simulink model "UIMUFSLR"  (R2022b)
settings: Solver=VariableStepAuto  StartTime=0.0  StopTime=10  RelTol=1e-3
values from neighbouring files (symbols this model uses):
  B1 = full(B{1,1})    [load_simulink_inputdata.m]
  B2 = full(B{1,2})    [load_simulink_inputdata.m]
  C1 = full(C{1,1})    [load_simulink_inputdata.m]
  C2 = full(C{1,2})    [load_simulink_inputdata.m]
  D1 = full(D{1,1})    [load_simulink_inputdata.m]
  D2 = full(D{1,2})    [load_simulink_inputdata.m]
  S1 = full(S{1,1})    [load_simulink_inputdata.m]
  S2 = full(S{1,2})    [load_simulink_inputdata.m]
  SC = SC + S{i}    [load_simulink_inputdata.m]
  XX1 = full(XX{1,1})    [load_simulink_inputdata.m]
  XX2 = full(XX{1,2})    [load_simulink_inputdata.m]
  Y = YT'    [load_simulink_inputdata.m]
undefined symbols (not defined in the file or in its folder): para
settings Model: Creator=86135  LastModifiedBy=86135

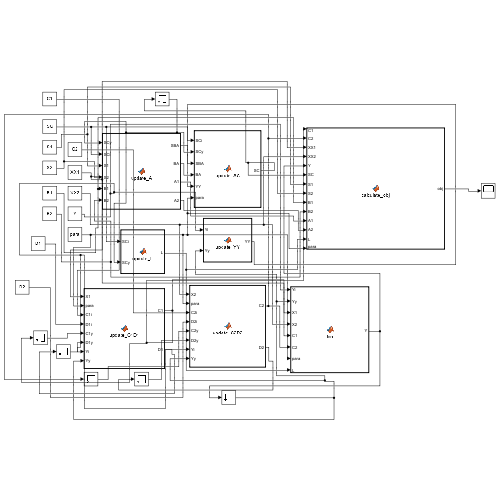
[thumbnail: Simulink's stored preview of the top-level diagram]
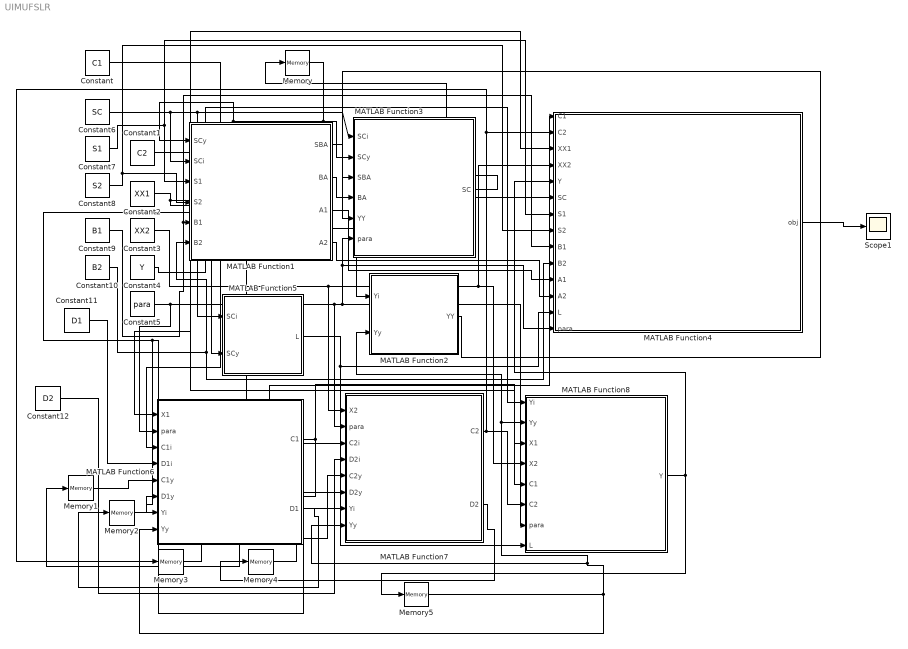
== system UIMUFSLR ==
  Constant : Constant  Value=C1
  Constant1 : Constant  Value=C2
  Constant10 : Constant  Value=B2
  Constant11 : Constant  Value=D1
  Constant12 : Constant  Value=D2
  Constant2 : Constant  Value=XX1
  Constant3 : Constant  Value=XX2
  Constant4 : Constant  Value=Y
  Constant5 : Constant  Value=para
  Constant6 : Constant  Value=SC
  Constant7 : Constant  Value=S1
  Constant8 : Constant  Value=S2
  Constant9 : Constant  Value=B1
  MATLAB Function1 : MATLAB Function  TreatAsAtomicUnit=on
  MATLAB Function2 : MATLAB Function  TreatAsAtomicUnit=on
  MATLAB Function3 : MATLAB Function  TreatAsAtomicUnit=on
  MATLAB Function4 : MATLAB Function  TreatAsAtomicUnit=on
  MATLAB Function5 : MATLAB Function  TreatAsAtomicUnit=on
  MATLAB Function6 : MATLAB Function  TreatAsAtomicUnit=on
  MATLAB Function7 : MATLAB Function  TreatAsAtomicUnit=on
  MATLAB Function8 : MATLAB Function  TreatAsAtomicUnit=on
  Memory : Memory  InitialCondition=ones(544,544)
  Memory1 : Memory  InitialCondition=ones(3183,5)
  Memory2 : Memory  InitialCondition=ones(3183,3183)
  Memory3 : Memory  InitialCondition=ones(3203,5)
  Memory4 : Memory  InitialCondition=ones(3203,3203)
  Memory5 : Memory  InitialCondition=ones(5,544)
  Scope1 : Scope
  wires:
  MATLAB Function4/1(obj) -> Scope1/1
  Constant/1 -> MATLAB Function6/3(C1i)
  Constant2/1 -> MATLAB Function8/3(X1), MATLAB Function4/3(XX1), MATLAB Function6/1(X1)
  Constant3/1 -> MATLAB Function8/4(X2), MATLAB Function4/4(XX2), MATLAB Function7/1(X2)
  Constant7/1 -> MATLAB Function4/7(S1), MATLAB Function1/3(S1)
  Constant8/1 -> MATLAB Function4/8(S2), MATLAB Function1/4(S2)
  MATLAB Function1/3(A1) -> MATLAB Function4/11(A1)
  MATLAB Function1/4(A2) -> MATLAB Function4/12(A2)
  Constant9/1 -> MATLAB Function1/5(B1), MATLAB Function4/9(B1)
  Constant10/1 -> MATLAB Function1/6(B2), MATLAB Function4/10(B2)
  Constant4/1 -> MATLAB Function8/1(Yi), MATLAB Function7/7(Yi), MATLAB Function6/7(Yi), MATLAB Function2/1(Yi)
  Constant5/1 -> MATLAB Function6/2(para), MATLAB Function8/7(para), MATLAB Function3/6(para), MATLAB Function4/14(para), MATLAB Function7/2(para)
  MATLAB Function1/1(SBA) -> MATLAB Function3/3(SBA)
  MATLAB Function1/2(BA) -> MATLAB Function3/4(BA)
  MATLAB Function2/1(YY) -> MATLAB Function3/5(YY)
  Constant6/1 -> MATLAB Function3/1(SCi), MATLAB Function5/1(SCi), MATLAB Function1/2(SCi)
  MATLAB Function3/1(SC) -> MATLAB Function4/6(SC), Memory/1
  MATLAB Function5/1(L) -> MATLAB Function4/13(L), MATLAB Function8/8(L)
  Memory/1 -> MATLAB Function5/2(SCy), MATLAB Function1/1(SCy), MATLAB Function3/2(SCy)
  Constant11/1 -> MATLAB Function6/4(D1i)
  MATLAB Function6/1(C1) -> Memory1/1, MATLAB Function4/1(C1), MATLAB Function8/5(C1)
  Memory1/1 -> MATLAB Function6/5(C1y)
  MATLAB Function6/2(D1) -> Memory2/1
  Memory2/1 -> MATLAB Function6/6(D1y)
  MATLAB Function7/1(C2) -> Memory3/1, MATLAB Function4/2(C2), MATLAB Function8/6(C2)
  MATLAB Function7/2(D2) -> Memory4/1
  Memory4/1 -> MATLAB Function7/6(D2y)
  Memory3/1 -> MATLAB Function7/5(C2y)
  Constant12/1 -> MATLAB Function7/4(D2i)
  Constant1/1 -> MATLAB Function7/3(C2i)
  MATLAB Function8/1(Y) -> MATLAB Function4/5(Y), Memory5/1
  Memory5/1 -> MATLAB Function7/8(Yy), MATLAB Function2/2(Yy), MATLAB Function8/2(Yy), MATLAB Function6/8(Yy)

== matlab function UIMUFSLR/MATLAB Function6 ==
  data: C1 output; X1 input; para input; D1 output; C1i input; D1i input; C1y input; D1y input; Yi input; Yy input
function [C1,D1]  = update_C1D1(X1,para,C1i,D1i,C1y,D1y,Yi,Yy)
alpha=para(1);
beta=para(2);
class_num=5;
% 定义 persistent 变量
persistent first_run;
if isempty(first_run)
    first_run = true;
end
if first_run
    C_u=X1*Yi'+beta*X1*X1'*C1i;
    C_d=X1*X1'*C1i+alpha*D1i*C1i+beta*(X1*X1')*C1i*ones(class_num,1)*ones(1,class_num);
    C1=C1i.*(pos(C_u)+neg(C_d))./max(pos(C_d)+neg(C_u),eps) ;
    tempD = 0.5 * (sqrt(sum(C1i.^2,2) + eps)).^(-1);
    D1 = diag(tempD);
    first_run = false;
else
    C_u=X1*Yy'+beta*X1*X1'*C1y;
    C_d=X1*X1'*C1y+alpha*D1y*C1y+beta*(X1*X1')*C1y*ones(class_num,1)*ones(1,class_num);
    C1=C1y.*(pos(C_u)+neg(C_d))./max(pos(C_d)+neg(C_u),eps) ;
    tempD = 0.5 * (sqrt(sum(C1.^2,2) + eps)).^(-1);
    D1 = diag(tempD);
end
 function result = pos(data)
        result =(abs(data)+data)/2;
    end
    function result = neg(data)
        result =(abs(data)-data)/2;
    end
end

== matlab function UIMUFSLR/MATLAB Function7 ==
  data: C2 output; X2 input; para input; D2 output; C2i input; D2i input; C2y input; D2y input; Yi input; Yy input
function [C2,D2]  = update_C2D2(X2,para,C2i,D2i,C2y,D2y,Yi,Yy)
alpha=para(1);
beta=para(2);
class_num=5;
% 定义 persistent 变量
persistent first_run;
if isempty(first_run)
    first_run = true;
end
if first_run
    C_u=X2*Yi'+beta*X2*X2'*C2i;
    C_d=X2*X2'*C2i+alpha*D2i*C2i+beta*(X2*X2')*C2i*ones(class_num,1)*ones(1,class_num);
    C2=C2i.*(pos(C_u)+neg(C_d))./max(pos(C_d)+neg(C_u),eps) ;
    tempD = 0.5 * (sqrt(sum(C2i.^2,2) + eps)).^(-1);
    D2 = diag(tempD);
    first_run = false;
else
    C_u=X2*Yy'+beta*X2*X2'*C2y;
    C_d=X2*X2'*C2y+alpha*D2y*C2y+beta*(X2*X2')*C2y*ones(class_num,1)*ones(1,class_num);
    C2=C2y.*(pos(C_u)+neg(C_d))./max(pos(C_d)+neg(C_u),eps) ;
    tempD = 0.5 * (sqrt(sum(C2.^2,2) + eps)).^(-1);
    D2 = diag(tempD);
end
 function result = pos(data)
        result =(abs(data)+data)/2;
    end
    function result = neg(data)
        result =(abs(data)-data)/2;
    end
end

== matlab function UIMUFSLR/MATLAB Function8 ==
  data: Y output; Yi input; Yy input; X1 input; X2 input; C1 input; C2 input; para input; L input
function Y  = fcn(Yi,Yy,X1,X2,C1,C2,para,L)
gamma=10000;
tau=para(3);
% 定义 persistent 变量
persistent first_run;
if isempty(first_run)
    first_run = true;
end
if first_run
    CTX=C1'*X1+C2'*X2;
    Y_u=CTX+2*gamma*Yi;
    Y_d=Yi+2*tau*Yi*L+2*gamma*Yi*Yi'*Yi;
    Y=Yi.*(pos(Y_u)+neg(Y_d))./max(pos(Y_d)+neg(Y_u),eps) ;
    Y = Y*diag(sqrt(1./(diag(Y'*Y)+eps)));
    first_run = false;
else
    CTX=C1'*X1+C2'*X2;
    Y_u=CTX+2*gamma*Yy;
    Y_d=Yy+2*tau*Yy*L+2*gamma*Yy*Yy'*Yy;
    Y=Yy.*(pos(Y_u)+neg(Y_d))./max(pos(Y_d)+neg(Y_u),eps) ;
    Y = Y*diag(sqrt(1./(diag(Y'*Y)+eps)));
end
 function result = pos(data)
        result =(abs(data)+data)/2;
    end
    function result = neg(data)
        result =(abs(data)-data)/2;
    end
end

== matlab function UIMUFSLR/MATLAB Function1 ==
  data: SBA output; SCy input; SCi input; S1 input; S2 input; BA output; A1 output; A2 output; B1 input; B2 input
function [SBA,BA,A1,A2] = update_A(SCy,SCi,S1,S2,B1,B2)
% 定义 persistent 变量
persistent first_run;
if isempty(first_run)
    first_run = true;
end
if first_run
    tem1=SCi-S1;
    tem2=SCi-S2;
    A1=diag(0.5./sqrt(sum(tem1.*tem1,1)+eps));
    A2=diag(0.5./sqrt(sum(tem2.*tem2,1)+eps));
    SBA=S1*B1*A1+S2*B2*A2;
    BA=B1*A1+B2*A2;
    first_run = false;
else
    tem1=SCy-S1;
    tem2=SCy-S2;
    A1=diag(0.5./sqrt(sum(tem1.*tem1,1)+eps));
    A2=diag(0.5./sqrt(sum(tem2.*tem2,1)+eps));
    SBA=S1*B1*A1+S2*B2*A2;
    BA=B1*A1+B2*A2;
end
end

== matlab function UIMUFSLR/MATLAB Function2 ==
  data: YY output; Yi input; Yy input
function YY  = update_YY(Yi,Yy)
% 定义 persistent 变量
persistent first_run;
if isempty(first_run)
    first_run = true;
end
if first_run
    a=Yi;
    b=Yi;
    if (size(a,1) == 1)%行为1时
        a = [a; zeros(1,size(a,2))];
        b = [b; zeros(1,size(b,2))];
    end

    aa=sum(a.*a); bb=sum(b.*b); ab=a'*b; %点乘，点乘自身相当于平方
    d = repmat(aa',[1 size(bb,2)]) + repmat(bb,[size(aa,2) 1]) - 2*ab;

    d = real(d);
    d = max(d,0);
    YY=d;
    first_run = false;
else
    a=Yy;
    b=Yy;
    if (size(a,1) == 1)%行为1时
        a = [a; zeros(1,size(a,2))];
        b = [b; zeros(1,size(b,2))];
    end

    aa=sum(a.*a); bb=sum(b.*b); ab=a'*b; %点乘，点乘自身相当于平方
    d = repmat(aa',[1 size(bb,2)]) + repmat(bb,[size(aa,2) 1]) - 2*ab;

    d = real(d);
    d = max(d,0);
    YY=d;
end
end

== matlab function UIMUFSLR/MATLAB Function3 ==
  data: SC output; SCi input; SCy input; SBA input; BA input; YY input; para input
function SC  = update_SC(SCi,SCy,SBA,BA,YY,para)
% 定义 persistent 变量
persistent first_run;
if isempty(first_run)
    first_run = true;
end
if first_run
    SC=SCi.*(pos(2*para(4)*SBA)+neg(2*para(4)*SCi*BA+para(3)*YY))./max(pos(2*para(4)*SCi*BA+para(3)*YY)+neg(2*para(4)*SBA),eps) ;
    SC=SC*diag(1./(sum(SC,1)+eps));
    first_run = false;
else
    SC=SCy.*(pos(2*para(4)*SBA)+neg(2*para(4)*SCy*BA+para(3)*YY))./max(pos(2*para(4)*SCy*BA+para(3)*YY)+neg(2*para(4)*SBA),eps) ;
    SC=SC*diag(1./(sum(SC,1)+eps));
end
    function result = pos(data)
        result =(abs(data)+data)/2;
    end
    function result = neg(data)
        result =(abs(data)-data)/2;
    end
end

== matlab function UIMUFSLR/MATLAB Function4 ==
  data: C1 input; C2 input; XX1 input; XX2 input; Y input; obj output; SC input; S1 input; S2 input; B1 input; B2 input; A1 input; A2 input; L input; para input
function obj  = calculate_obj(C1,C2,XX1,XX2,Y,SC,S1,S2,B1,B2,A1,A2,L,para)

class_num=5;
obj=norm(C1'*XX1-Y,'fro').^2+para(4)*trace((SC-S1)*B1*A1*(SC'-S1'))+para(1).*sum((sum((C1).^2,2)).^(1/2))+para(2)*trace(XX1'*C1*ones(class_num,1)*ones(1,class_num)*C1'*XX1-XX1'*C1*C1'*XX1);
obj=obj+norm(C2'*XX2-Y,'fro').^2+para(4)*trace((SC-S2)*B2*A2*(SC'-S2'))+para(1).*sum((sum((C2).^2,2)).^(1/2))+para(2)*trace(XX2'*C2*ones(class_num,1)*ones(1,class_num)*C2'*XX2-XX2'*C2*C2'*XX2);
obj=obj+para(3)*trace(Y*L*Y');

end

== matlab function UIMUFSLR/MATLAB Function5 ==
  data: L output; SCi input; SCy input
function L  = update_L(SCi,SCy)
% 定义 persistent 变量
persistent first_run;
if isempty(first_run)
    first_run = true;
end
if first_run
    tem = diag( sum( (SCi + SCi.')/2 ) );
    L = tem - (SCi + SCi')/2 ;
    first_run = false;
else
    tem = diag( sum( (SCy + SCy.')/2 ) );
    L = tem - (SCy + SCy')/2 ;
end
end
